simulink model "MPC_Validation"  (R2020a)
settings: Solver=FixedStepAuto  StartTime=0.0  StopTime=tsim  FixedStep=baseRate  RelTol=1e-3  EnableMultiTasking=on
values from neighbouring files (symbols this model uses):
  Ad = -C(7:12,4:9)    [theFastMPCSolver3.m]    (also in theInitializer.m = dss.A)
  ALGORITHM = 5    [Run_Initializer.m]
  baseRate = 0.05    [Run_Initializer.m]
  cdockdeltax = rc+rt-2*dockoffset    (= 0.165)    [theInitializer.m]
  cdockoa = atan(cdockdeltay/cdockdeltax)    [theInitializer.m]
  Cmat = zeros(6*N,9*N)    [theInitializer.m]
  con0 = [n*N, 2*N, N, N, N]    [Run_Initializer.m]
  drop_states_ARM = [ pi/2, pi/2, 0]    [Run_Initializer.m]
  drop_states_BLACK = rand([1,3])/10+init_states_BLACK    [Run_Initializer.m]
  drop_states_BLUE = rand([1,3])/10+init_states_BLUE    [Run_Initializer.m]
  drop_states_RED = rand([1,3])/10+init_states_RED    [Run_Initializer.m]
  ecoa = pi/2    (= 1.57079632679)    [theInitializer.m]
  F_Black_X_nominal = 0.2196    [Run_Initializer.m]
  F_Black_Y_nominal = 0.2825    [Run_Initializer.m]
  F_Blue_X_nominal = 0.2196    [Run_Initializer.m]
  F_Blue_Y_nominal = 0.2825    [Run_Initializer.m]
  F_red_X_nominal = 0.2196    [Run_Initializer.m]
  F_red_Y_nominal = 0.2825    [Run_Initializer.m]
  F_thrusters_BLACK = [F_Black_X_nominal; F_Black_X_nominal;                             F_Black_Y_nominal; F_Black_Y_nominal; F_Black_X_nominal;                              F_Black_X_nominal; F_Black_Y_nominal; F_Black_Y_nominal]    [Run_Initializer.m]
  F_thrusters_BLUE = [F_Blue_X_nominal; F_Blue_X_nominal;                             F_Blue_Y_nominal; F_Blue_Y_nominal; F_Blue_X_nominal;                              F_Blue_X_nominal; F_Blue_Y_nominal; F_Blue_Y_nominal]    [Run_Initializer.m]
  F_thrusters_RED = [F_red_X_nominal; F_red_X_nominal;                             F_red_Y_nominal; F_red_Y_nominal; F_red_X_nominal;                              F_red_X_nominal; F_red_Y_nominal; F_red_Y_nominal]    [Run_Initializer.m]
  Fmat = reshape(repmat([umax,umax,taumax],N,1),3*N,1)    [theInitializer.m]
  gamma = 0.95    [theInitializer.m]
  Gamma1 = 0.0025    [Run_Initializer.m]
  Gamma2 = 100    [Run_Initializer.m]
  Gamma3 = 10    [Run_Initializer.m]
  Gamma4 = 0.001    [Run_Initializer.m]
  Gamma5 = 100    [Run_Initializer.m]
  Gamma6 = 0.001    [Run_Initializer.m]
  H = blkdiag(pattern{:})    [theInitializer.m]
  home_states_BLACK = [ xLength/2, yLength/2, 0]    [Run_Initializer.m]
  home_states_BLUE = [ xLength/2-0.9, yLength/2+0.5, 0]    [Run_Initializer.m]
  home_states_RED = [ xLength/2+0.7, yLength/2, pi]    [Run_Initializer.m]
  init_states_BLACK = [ct;thetat0].'    [Run_Initializer.m]
  init_states_BLUE = [pobj1;0].'    [Run_Initializer.m]
  init_states_RED = xi(1:3).'    [Run_Initializer.m]
  isCONTROL = 0    [Run_Initializer.m]
  Kd_elarm = 0.05    [Run_Initializer.m]
  Kd_sharm = 0.05    [Run_Initializer.m]
  Kd_tb = 0.4    [Run_Initializer.m]
  Kd_tblue = 0.4    [Run_Initializer.m]
  Kd_tr = 0.4    [Run_Initializer.m]
  Kd_wrarm = 0.005    [Run_Initializer.m]
  Kd_xb = 8    [Run_Initializer.m]
  Kd_xblue = 8    [Run_Initializer.m]
  Kd_xr = 8    [Run_Initializer.m]
  Kd_yb = 8    [Run_Initializer.m]
  Kd_yblue = 8    [Run_Initializer.m]
  Kd_yr = 8    [Run_Initializer.m]
  KOZ_actual = KOZ + rc*sqrt(2)*1.1    [theInitializer.m]
  Kp = [0.08 0 0 ... (first row only)    [Run_Initializer.m]
  Kp_elarm = 0.08    [Run_Initializer.m]
  Kp_sharm = 0.15    [Run_Initializer.m]
  Kp_tb = 0.1    [Run_Initializer.m]
  Kp_tblue = 0.1    [Run_Initializer.m]
  Kp_tr = 0.1    [Run_Initializer.m]
  Kp_wrarm = 0.007    [Run_Initializer.m]
  Kp_xb = 2    [Run_Initializer.m]
  Kp_xblue = 2    [Run_Initializer.m]
  Kp_xr = 2    [Run_Initializer.m]
  Kp_yb = 2    [Run_Initializer.m]
  Kp_yblue = 2    [Run_Initializer.m]
  Kp_yr = 2    [Run_Initializer.m]
  Kv = [0.05 0 0 ... (first row only)    [Run_Initializer.m]
  maxiterations = 10    [Run_Initializer.m]
  N = 15    [Run_Initializer.m]    (also in theFastMPCSolver2.m = length(z)/9; theFastMPCSolver3.m = length(z)/9)
  n = size(b,1)    [my_fbsubstitution.m]    (also in theFastMPCSolver3.m)
  noise_variance_BLACK = 0    [Run_Initializer.m]
  noise_variance_BLUE = 0    [Run_Initializer.m]
  noise_variance_RED = 0    [Run_Initializer.m]
  noisemean = 0.1    [Run_Initializer.m]
  pdockoa = atan(rt/cdockdeltax)    [theInitializer.m]
  pdockr = sqrt(cdockdeltax*cdockdeltax + rt*rt)    [theInitializer.m]
  Phase0_End = Phase0_Duration    (= 5)    [Run_Initializer.m]
  Phase1_End = Phase0_Duration + Phase1_Duration    (= 10)    [Run_Initializer.m]
  Phase2_End = Phase0_Duration + Phase1_Duration +                                   Phase2_Duration    (= 36)    [Run_Initializer.m]
  Phase3_End = Phase0_Duration + Phase1_Duration +                                   Phase2_Duration + Phase3_Duration    (= 166)    [Run_Initializer.m]
  Phase3_SubPhase1_End = Phase2_End + Phase3_SubPhase1_Duration    (= 40)    [Run_Initializer.m]
  Phase3_SubPhase2_End = Phase2_End + Phase3_SubPhase1_Duration +                                   Phase3_SubPhase2_Duration    (= 42)    [Run_Initializer.m]
  Phase3_SubPhase3_End = Phase2_End + Phase3_SubPhase1_Duration +                                   Phase3_SubPhase2_Duration +                                  Phase3_SubPhase3_Duration    (= 44)    [Run_Initializer.m]
  Phase3_SubPhase4_End = Phase2_End + Phase3_SubPhase1_Duration +                                   Phase3_SubPhase2_Duration +                                  Phase3_SubPhase3_Duration +                                  Phase3_SubPhase4_Duration    [Run_Initializer.m]
  Phase4_End = Phase0_Duration + Phase1_Duration +                                   Phase2_Duration + Phase3_Duration +                                   Phase4_Duration    (= 186)    [Run_Initializer.m]
  Phase5_End = Phase0_Duration + Phase1_Duration +                                   Phase2_Duration + Phase3_Duration +                                   Phase4_Duration + Phase5_Duration    (= 191)    [Run_Initializer.m]
  rcone = 0.75    [theInitializer.m]
  rdock = sqrt(cdockdeltax*cdockdeltax + cdockdeltay*cdockdeltay)    [theInitializer.m]
  serverRate = 0.1    [Run_Initializer.m]
  Sj = [KOZ_actual^(-2),0; 0,KOZ_actual^(-2)]    [theInitializer.m]
  taumax = umax*rc    (= 0.0225)    [theInitializer.m]
  Td = 2    [Run_Initializer.m]
  thetah = 20.0 * d2r    (= 0.349065850399)    [theInitializer.m]
  thetat_dot = 0 * d2r    (= 0)    [Run_Initializer.m]
  thruster_dist2CG_BLACK = [83.42;-52.58;55.94;-60.05;54.08;-53.92;77.06;-55.94]    [Run_Initializer.m]
  thruster_dist2CG_BLUE = [73.54;-64.46;81.39;-60.11;64.46;-65.94;54.61;-74.39]    [Run_Initializer.m]
  thruster_dist2CG_RED = [49.92;-78.08;70.46;-63.54;81.08;-50.42;57.44;-75.96]    [Run_Initializer.m]
  tol = 0.00015    [Run_Initializer.m]
  Tz_lim_elarm = .1    (= 0.1)    [Run_Initializer.m]
  Tz_lim_sharm = .1    (= 0.1)    [Run_Initializer.m]
  Tz_lim_wrarm = .1    (= 0.1)    [Run_Initializer.m]
  Umat = zeros(3*N,9*N)    [theInitializer.m]
  umax = 0.15    [theInitializer.m]
  vobj1 = [0.00;0.00]    [Run_Initializer.m]
  vtar = [0.0;0.0]    [Run_Initializer.m]
undefined symbols (not defined in the file or in its folder): DiscIntNeverNeededParam, model_param, platformSelection, simMode, WhoAmI
libraries: dspstat3 x23, dspsigops x15, embdlinuxlib x10, raspberrypiBasiclib x10, simulink x8, MainLibrary x7, mspfiltlib x3, dsparch4 x3, dspswit3 x2, sensehatlib x1
(part 16 of 18)

== matlab function MPC_Validation/Triggered Subsystem/If Action Subsystem1/MPC ==
  data: CONTROL output; xi input; Td parameter; N parameter; pdockr parameter; rdock parameter; thetah parameter; KOZ_actual parameter; Sj parameter; rcone parameter; Ad parameter; con0 parameter; Cmat parameter; Umat parameter; Fmat parameter; H parameter; gamma parameter; tol parameter; x0 output; rhold output; x0 input; rhold input; ALGORITHM parameter; umax parameter; taumax parameter; n parameter; ct input; pobj1 input; vtar input; vobj1 input; thetat0 input; thetat_dot input; pdockoa parameter; ecoa parameter; cdockoa parameter; maxiterations parameter; CPUTIME output; cdockdeltax parameter
function [CONTROL, x0, rhold, CPUTIME] = MPC(xi,Td, N, pdockr, rdock, thetah, KOZ_actual, Sj, rcone, Ad, con0, Cmat, Umat, Fmat, H, gamma, tol, x0, rhold, ALGORITHM, umax, taumax, n, ct, pobj1, vtar, vobj1, thetat0, thetat_dot, pdockoa, ecoa, cdockoa, maxiterations, cdockdeltax)
    % COPY-PASTED FROM LOOP IN MAIN
    d2r = pi/180;
    
    N = 15;
    maxiterations = 10;
    
    % The moving target and obstacle positions for the current sampling instant, k
    [pobj1hz, ptar] = theMovingObstacleHorizonParameters(Td,N,ct,pobj1,vtar,vobj1);
    
    % The rotating target parameters for the current sampling instant, k
    [thetat,m1,m2,nc1,nc2,pdock,xt,cdock] = theRotatingTargetHorizonParameters(Td,N,ptar,vtar,pdockr,rhold,rdock,cdockoa,pdockoa,ecoa,thetat_dot,thetah,thetat0,cdockdeltax);
    
    % Reshape the xt variable for use in theObjectiveFunction, ignore the
    % current state and reform into [03 xt(2) 03 xt(2) 03 ... 03 xt(N+1)]
    xt9 = zeros(9,N);
    xt9(4:9,:) = xt(:,2:N+1);
    xt9 = reshape(xt9, [9*N,1]);
    
    % The reference trajectory of the chaser over the horizon of instant k
    pxref = theReferenceTrajectory(x0,N); % 2xN

    % The points ro on the KOZ boundaries of the obstacles over the horizon
    ro_1 = theObstacleLinearizer(pxref,pobj1hz(:,2:N+1),KOZ_actual);
    ro_t = theObstacleLinearizer(pxref,ptar(:,2:N+1),rhold);
    
    % Reshape pdock for use in the linearized matrix constraints
    pdock9 = zeros(9,N);
    pdock9(4:5,:) = pdock(:,2:N+1);
    pdock9 = reshape(pdock9, [9*N,1]);

    % Make the ro_X and robj9 vectors for obstacle constraints
    ro_1_9 = zeros(9,N);
    ro_1_9(4:5,:) = ro_1;
    ro_1_9 = reshape(ro_1_9,9*N,1);

    ro_t_9 = zeros(9,N);
    ro_t_9(4:5,:) = ro_t;
    ro_t_9 = reshape(ro_t_9,9*N,1);

    robj1_9 = zeros(9,N);
    robj1_9(4:5,:) = pobj1hz(:,2:N+1);
    robj1_9 = reshape(robj1_9,9*N,1);

    rtar_9 = zeros(9,N);
    rtar_9(4:5,:) = ptar(:,2:N+1);
    rtar_9 = reshape(rtar_9,9*N,1);

    % Make the matrix for obstacle constraints
    S1 = Sj;
    St = [1/(rhold*rhold), 0; 0, 1/(rhold*rhold)];

    E1 = (ro_1 - pobj1hz(:,2:N+1)).' * S1;
    Et = (ro_t - ptar(:,2:N+1)).' * St;

    D1 = zeros(N,(9*N));
    Dt = zeros(N,(9*N));
    for row = 1:N
        D1(row,4+(row-1)*9:5+(row-1)*9) = E1(row,:);
        Dt(row,4+(row-1)*9:5+(row-1)*9) = Et(row,:);
    end  
    
    % Define the b vector for Cx = b dynamics constraint
    bvec = zeros(6*N,1);
    bvec(1:6) = Ad*xi;
    
    % Define arrays for the hyperplane normal arrays to be used for the entry cone constraints
    nc1m = zeros(N,9*N);
    nc2m = zeros(N,9*N);
        
    % Determine if the entry cone constraints should be on
    if ((xi(1:2) - cdock(1:2,1)).' * (xi(1:2) - cdock(1:2,1)) < rcone*rcone) % if chaser is within rcone range
        
        temp1 = -nc1(2,:) * x0(4:5) + nc1(2,:) * pdock9(4:5);
        temp2 = nc2(2,:) * x0(4:5) - nc2(2,:) * pdock9(4:5);
        
              
        if temp1 <= 0 && temp2 <= 0 % only turn ec constraints on if it won't cause infeasibilities at the next step
            
        
            withEntryCone = 1; % turn on
            con = [n*N, 2*N, N, N, N, N, N];

            % Create Nx2N matrix of the entry cone normal to each hyperplane
            % Should be in the form
            % ncm = [ 0_1x3 n1_1x2 0_1x4 0_1x3  0_1x2 0_1x4  ... 0_1x3 0_1x2 0_1x4
            %         0_1x3  0_1x2 0_1x4 0_1x3 n2_1x2 0_1x4  ... 0_1x3 0_1x2 0_1x4
            %                           ...
            %         0_1x3  0_1x2 0_1x4 0_1x3  0_1x2 0_1x4  ... 0_1x3 nN+1_1x2 0_1x4
            for i=1:N
                nc1m(i,4+(i-1)*9:5+(i-1)*9) = nc1(i+1,:);
                nc2m(i,4+(i-1)*9:5+(i-1)*9) = nc2(i+1,:);
            end
        else
            
            withEntryCone = 0; % turn off
            con = con0;

            % FOR PLOTTING PURPOSES
            m1 = NaN;
            m2 = NaN;
        end
                
    else
        withEntryCone = 0; % turn off
        con = con0;
        
        % FOR PLOTTING PURPOSES
        m1 = NaN;
        m2 = NaN;
    end
    

    
%     if ALGORITHM == 5     
        % Constraint Matrix
        if ~withEntryCone
            Wmat = [-2*D1;-2*Dt];
        else
            Wmat = [-2*D1;-2*Dt;-nc1m;nc2m];
        end
%     % THIS NEEDS TO BE CLEANED UP
%     elseif ALGORITHM == 6 || ALGORITHM == 7
%         if withEntryCone
%             Wmat = zeros(10*N,9*N);
%             hvec = zeros(10*N,1);
%         else
%             Wmat = zeros(8*N,9*N);
%             hvec = zeros(8*N,1);
%         end
% 
%         for index = 0:N-1
%             blockc = 9*index;
%             if withEntryCone
%                 blockr = 10*index;
%                 Wmat(9+blockr,:) = -nc1m(index+1,:);
%                 Wmat(10+blockr,:) = nc2m(index+1,:);
%             else
%                 blockr = 8*index;
%             end
%             Wmat(1+blockr:3+blockr,1+blockc:3+blockc) = eye(3);
%             Wmat(4+blockr:6+blockr,1+blockc:3+blockc) = -eye(3);
%             Wmat(7+blockr,:) = -2*D1(index+1,:);
%             Wmat(8+blockr,:) = -2*Dt(index+1,:);
%         end
% 
%         f_D1 = -ones(N,1) - D1*(ro_1_9 + robj1_9);
%         f_Dt = -ones(N,1) - Dt*(ro_t_9 + rtar_9);   
%         if withEntryCone % if entry cone constraints turned on
%             f_ec1 = -nc1m * pdock9;
%             f_ec2 = nc2m * pdock9;
%         end
% 
%         for index = 0:N-1
%             if withEntryCone % if entry cone constraints turned on
%                 blockr = 10*index;
%                 hvec(9+blockr) = f_ec1(index+1);
%                 hvec(10+blockr) = f_ec2(index+1);
%             else
%                 blockr = 8*index;
%             end
% 
%             hvec(1+blockr:3+blockr) = [umax;umax;taumax];
%             hvec(4+blockr:6+blockr) = [umax;umax;taumax];
%             hvec(7+blockr) = f_D1(index+1);
%             hvec(8+blockr) = f_Dt(index+1);
%         end
% 
%     end
    
    % Constraint upper and lower limits
%     if ALGORITHM == 5
        [cl,cu,bineqvec] = theConstraintLimits4(Umat,Fmat,Wmat,con0,con,...
            D1,Dt,ro_1_9,ro_t_9,robj1_9,rtar_9,nc1m,...
            nc2m,pdock9);
%     end
    
    

%     
%     % Ensure a feasible start
%     if ALGORITHM == 6 || ALGORITHM == 7
%         if any((hvec - Wmat*x0) <= 0)
%             disp('Started with infeasible solution (outside).');
%             infeas0 = find((hvec - Wmat*x0) <= 0);
%             disp(infeas0)
% 
%             % Find a new feasible z-val for the violated constraint(s)
%             for ind = infeas0.'
%                 if size(con) == size(con0) % no ec constraints yet
%                     ind_startrange = 7 + 8*idivide(ind,int16(8+1));
%                     ind_endrange = ind_startrange + 1;
%                 else
%                     ind_startrange = 7 + 10*idivide(ind,int16(10+1));
%                     ind_endrange = ind_startrange + 3;
%                 end
% %                 disp(ind_startrange)
% %                 disp(ind_endrange)
%                     
%                 z_infeas_ind = find(Wmat(ind,:)); % optimization variable(s) to vary
%     %             disp('z(infeas)=')
%     %             disp(z_infeas_ind)
% 
%                 newind = z_infeas_ind - 9;
%                 
%                 search_range = 1;
%                 search_stepnum = 1001;
%                 
%                 while (1)
%                     if newind < 0
%                         disp("Sampling...")
% 
%                         % make a grid of search points
%                         try_x = linspace(x0(z_infeas_ind(1))-search_range,x0(z_infeas_ind(1))+search_range,search_stepnum);
%                         try_y = linspace(x0(z_infeas_ind(2))-search_range,x0(z_infeas_ind(2))+search_range,search_stepnum);
%                         [xx,yy] = meshgrid(try_x,try_y);
% 
%                         % calcuate the constraint at each grid point
% %                         temp = zeros(search_stepnum,search_stepnum);
%                         temp2 = zeros(search_stepnum*search_stepnum,3);
%                         for i1=1:search_stepnum
%                             for i2 = 1:search_stepnum
%                                 temp = hvec(ind_startrange:ind_endrange) - Wmat(ind_startrange:ind_endrange,z_infeas_ind)*[xx(i1,i2);yy(i1,i2)];
% 
%                                 % take note of grid points that satisfy the constraint
%                                 if ~any(temp <= 0)
%                                     temp2((i1-1)*search_stepnum+i2,1) = min(temp);
%                                     temp2((i1-1)*search_stepnum+i2,2) = i1;
%                                     temp2((i1-1)*search_stepnum+i2,3) = i2;
%                                 end
%                             end
%                         end
% 
%                         % get rid of data that does not satisfy the constraints
%                         temp2( ~any(temp2,2), : ) = [];  %rows
%                         
%                         if isempty(temp2)
%                             search_range = 3;
%                             search_stepnum = search_stepnum * 2;
%                             continue
%                         end
% 
%                         % choose one of the grid points that satisfy the constraint
%                         % currently finds the first minimum value... could be further improved
%                         ind_of_min = find(temp2(:,1) == min(temp2(:,1)));
%                         ind_chosen = ind_of_min(1);
% 
%                         % update the x0 with the new grid point
%                         [i1i2_chosen] = temp2(ind_chosen,[2,3]);
%                         i1_chosen = i1i2_chosen(1);
%                         i2_chosen = i1i2_chosen(2);
%                         x0(z_infeas_ind) = [xx(i1_chosen,i2_chosen);yy(i1_chosen,i2_chosen)];                     
%                         
%                     else
%                         x0(z_infeas_ind) = x0(newind); % re-tracing previous sol'n
%                     end
% 
%                     if (hvec(ind)- Wmat(ind,:)*x0) <= 0
%                         if newind < 0
%                             disp("Solution not in sample range.")
%                         else
%                             newind = newind - 9;
%                         end
%                     else
%                         disp("Resolved.")
%                         break
%                         
%                     end
%                 end
%             end
%         end
%        
%     end
%     
%     
%     
%     % Setup Options
%     if ALGORITHM == 5
        options = optimoptions('quadprog','Algorithm','active-set','MaxIterations',10);
%     elseif ALGORITHM == 6 || ALGORITHM == 7
%         nu = zeros(6*N,1);
%     end
%     
%     % Solve!
%     if ALGORITHM == 5
        tic
        [x,fval] = quadprog(H,-H.'*xt9,Wmat,bineqvec,Cmat,bvec,cl,cu,x0,options);
        CPUTIME = toc;
%     elseif ALGORITHM == 6
%         disp('----------------------------------------------')
%         disp(string(count))
%         
%         tic
%         [x,nu] = theFastMPCSolver2(x0,nu,xt9,H,Cmat,bvec,Wmat,hvec,1e-9,0.01,0.95,maxiterations);
%         solCPUtime = toc;
%     elseif ALGORITHM == 7
%         disp('----------------------------------------------')
%         disp(string(count))
%         tic
%         [x,nu] = theFastMPCSolver3(x0,nu,xt9,H,Cmat,bvec,Wmat,hvec,1e-9,0.01,0.95,maxiterations);
%         solCPUtime = toc;
%     end
   

    % Save data
%     sol(end+1:end+9) = x(1:9);
%     soliter(1:n,count) = xi;
%     soliter(n+1:n+9*N,count) = x;
%     solpobj(count,1) = pobj1hz(1,1); 
%     solpobj(count,2) = pobj1hz(2,1);
%     solpobj(count,3) = pobj2hz(1,1);
%     solpobj(count,4) = pobj2hz(2,1);
%     solptar(count,1) = ptar(1,1);
%     solptar(count,2) = ptar(2,1);
%     solm1(count,1) = m1(1);
%     solm2(count,1) = m2(1);
%     solthetat(count,1) = thetat(1);
%     solpdock(count,1:2) = pdock(:,1);
%     if ALGORITHM == 0
%         solJ(end+1) = theObjectiveFunction0(x,N,xt,P,Q,R);
%     elseif ALGORITHM > 0
%         solJ(end+1) = theObjectiveFunction123(x,xt9,H);
%     end
%     count = count + 1;

    CONTROL = x(1:3);
    
    % Determine if the chaser is docked using the 'current' positions of
    % the chaser and docking condition; done using only position
    if (xi(1:2) - cdock(1:2,1)).' * (xi(1:2) - cdock(1:2,1)) < tol
        isdocked = 1;
    end
    
    % Set the next guess as the solution from the previous iteration
    xi = x(4:9); % the next 'current' state of the chaser spacecraft
    % x0 = [x(10:end);0;0;0;Ad*x0(4+9*(N-2):9+9*(N-2)) + Bd*x0(1+9*(N-1):3+9*(N-1))];
    x0 = [x(10:end);0;0;0;x(4+9*(N-1):9+9*(N-1))];
    
    % Update rhold if:
    %  - the position of the chaser matches the holding position, within tolerance
    %  - the attitude of the chaser matches the docking condition, within tolerance
    %  - the holding radius is larger than its minimum allowable size, rdock
    if abs((xi(1:2) - xt(1:2,1)).' * (xi(1:2) - xt(1:2,1))) < 0.5 % if position error is below tolerance
        if abs(xi(3) - cdock(3,1)) < 10*d2r % if attitude error is below tolerance
            if rhold > rdock
                rhold = rhold * gamma; % decrease the holding radius
                if rhold < rdock
                    rhold = rdock; % set to the minimum holding radius, rdock
                end
            end
        end
    end
    
    % Set the next 'current' target and obstacle positions
%     ct = ptar(:,2);
%     pobj1 = pobj1hz(:,2); 
%     pobj2 = pobj2hz(:,2);
        
    % Set the new target theta value for the next iteration
%     thetat0 = thetat(2);
    
end

== matlab function MPC_Validation/Phase #3: Experiment/Change BLACK Behavior/Sub-Phase #2 /Hough Control/MATLAB Function2 ==
  data: Oy output; z input; Ox output
function [Oy, Ox]   = C3( z )
%C3 gives the rotation matrix about the z-axis for an angle 'z'
%   z - the angle about the z-axis which you rotate
%   A - the rotation matrix

Ox = [cos(z) sin(z); -sin(z) cos(z)]*[1;0];
Oy = [cos(z) sin(z); -sin(z) cos(z)]*[0;1];
end

== matlab function MPC_Validation/Phase #3: Experiment/Change BLACK Behavior/Sub-Phase #2 /Hough Control/MATLAB Function4 ==
  data: Oy input; e_out output; e_in input
function e_out = fcn(Oy, e_in)

a = sign(Oy'*e_in);
e_out = -a*norm(e_in);

== matlab function MPC_Validation/Phase #3: Experiment/Change BLACK Behavior/Sub-Phase #4/Hough Control/MATLAB Function4 ==
  data: Oy input; e_out output; e_in input
function e_out = fcn(Oy, e_in)

a = sign(Oy'*e_in);
e_out = -a*norm(e_in);

== matlab function MPC_Validation/Phase #3: Experiment/Change BLACK Behavior/Sub-Phase #1/Hough Control/MATLAB Function2 ==
  data: Oy output; z input; Ox output
function [Oy, Ox]   = C3( z )
%C3 gives the rotation matrix about the z-axis for an angle 'z'
%   z - the angle about the z-axis which you rotate
%   A - the rotation matrix

Ox = [cos(z) sin(z); -sin(z) cos(z)]*[1;0];
Oy = [cos(z) sin(z); -sin(z) cos(z)]*[0;1];
end

== matlab function MPC_Validation/Phase #3: Experiment/Change BLACK Behavior/Sub-Phase #1/Hough Control/MATLAB Function3 ==
  data: z input; Ox output
function Ox    = C3( z )
%C3 gives the rotation matrix about the z-axis for an angle 'z'
%   z - the angle about the z-axis which you rotate
%   A - the rotation matrix

Ox = [cos(z) sin(z); -sin(z) cos(z)]*[1;0];
end

== matlab function MPC_Validation/Phase #3: Experiment/Change BLACK Behavior/Sub-Phase #1/Hough Control/MATLAB Function4 ==
  data: Oy input; e_out output; e_in input
function e_out = fcn(Oy, e_in)

a = sign(Oy'*e_in);
e_out = -a*norm(e_in);

== matlab function MPC_Validation/Phase #3: Experiment/Change BLUE Behavior/Sub-Phase #4/Hough Control/MATLAB Function3 ==
  data: z input; Ox output
function Ox    = C3( z )
%C3 gives the rotation matrix about the z-axis for an angle 'z'
%   z - the angle about the z-axis which you rotate
%   A - the rotation matrix

Ox = [cos(z) sin(z); -sin(z) cos(z)]*[1;0];
end

== matlab function MPC_Validation/Phase #3: Experiment/Change BLUE Behavior/Sub-Phase #4/Hough Control/MATLAB Function4 ==
  data: Oy input; e_out output; e_in input
function e_out = fcn(Oy, e_in)

a = sign(Oy'*e_in);
e_out = -a*norm(e_in);

== matlab function MPC_Validation/Phase #5: Hold Home/Change BLACK Behavior/Hough Control/MATLAB Function2 ==
  data: Oy output; z input; Ox output
function [Oy, Ox]   = C3( z )
%C3 gives the rotation matrix about the z-axis for an angle 'z'
%   z - the angle about the z-axis which you rotate
%   A - the rotation matrix

Ox = [cos(z) sin(z); -sin(z) cos(z)]*[1;0];
Oy = [cos(z) sin(z); -sin(z) cos(z)]*[0;1];
end

== matlab function MPC_Validation/Phase #5: Hold Home/Change BLACK Behavior/Hough Control/MATLAB Function3 ==
  data: z input; Ox output
function Ox    = C3( z )
%C3 gives the rotation matrix about the z-axis for an angle 'z'
%   z - the angle about the z-axis which you rotate
%   A - the rotation matrix

Ox = [cos(z) sin(z); -sin(z) cos(z)]*[1;0];
end

== matlab function MPC_Validation/Phase #5: Hold Home/Change BLACK Behavior/Hough Control/MATLAB Function4 ==
  data: Oy input; e_out output; e_in input
function e_out = fcn(Oy, e_in)

a = sign(Oy'*e_in);
e_out = -a*norm(e_in);

== matlab function MPC_Validation/Phase #4: Return Home/Change BLUE Behavior/Hough Control/MATLAB Function2 ==
  data: Oy output; z input; Ox output
function [Oy, Ox]   = C3( z )
%C3 gives the rotation matrix about the z-axis for an angle 'z'
%   z - the angle about the z-axis which you rotate
%   A - the rotation matrix

Ox = [cos(z) sin(z); -sin(z) cos(z)]*[1;0];
Oy = [cos(z) sin(z); -sin(z) cos(z)]*[0;1];
end

== matlab function MPC_Validation/Phase #4: Return Home/Change BLUE Behavior/Hough Control/MATLAB Function3 ==
  data: z input; Ox output
function Ox    = C3( z )
%C3 gives the rotation matrix about the z-axis for an angle 'z'
%   z - the angle about the z-axis which you rotate
%   A - the rotation matrix

Ox = [cos(z) sin(z); -sin(z) cos(z)]*[1;0];
end

== matlab function MPC_Validation/Phase #4: Return Home/Change BLUE Behavior/Hough Control/MATLAB Function4 ==
  data: Oy input; e_out output; e_in input
function e_out = fcn(Oy, e_in)

a = sign(Oy'*e_in);
e_out = -a*norm(e_in);

== matlab function MPC_Validation/Simulate Plant Dynamics/BLUE Dynamics/BLUE  Dynamics Model/MATLAB Function ==
  data: control_inputs input; x_ddot output; model_param parameter
function x_ddot = BLUE_dynamics(control_inputs, model_param)

%#codegen
% Fully define the size of x_ddot() for code generation:
x_ddot     = zeros(3,1);

% Extract the servicer model parameters from the model_param vector defined
% in initialize.m:
m_BLUE    = model_param(5);
I_BLUE    = model_param(6);

% Extract the control inputs from the control_input vector:
Fx        = control_inputs(1);              % [N]
Fy        = control_inputs(2);              % [N]
Tz        = control_inputs(3);              % [N.m]

% Calculate the state acceleration vector:
x_ddot(1) = Fx/m_BLUE;                      % [m/s^2]
x_ddot(2) = Fy/m_BLUE;                      % [m/s^2]
x_ddot(3) = Tz/I_BLUE;                      % [rad/s^2]

end

== matlab function MPC_Validation/Phase #3: Experiment/Change BLUE Behavior/Sub-Phase #2 /Hough Control/MATLAB Function2 ==
  data: Oy output; z input; Ox output
function [Oy, Ox]   = C3( z )
%C3 gives the rotation matrix about the z-axis for an angle 'z'
%   z - the angle about the z-axis which you rotate
%   A - the rotation matrix

Ox = [cos(z) sin(z); -sin(z) cos(z)]*[1;0];
Oy = [cos(z) sin(z); -sin(z) cos(z)]*[0;1];
end

== matlab function MPC_Validation/Phase #3: Experiment/Change BLUE Behavior/Sub-Phase #2 /Hough Control/MATLAB Function3 ==
  data: z input; Ox output
function Ox    = C3( z )
%C3 gives the rotation matrix about the z-axis for an angle 'z'
%   z - the angle about the z-axis which you rotate
%   A - the rotation matrix

Ox = [cos(z) sin(z); -sin(z) cos(z)]*[1;0];
end

== matlab function MPC_Validation/Phase #3: Experiment/Change BLUE Behavior/Sub-Phase #2 /Hough Control/MATLAB Function4 ==
  data: Oy input; e_out output; e_in input
function e_out = fcn(Oy, e_in)

a = sign(Oy'*e_in);
e_out = -a*norm(e_in);

== matlab function MPC_Validation/Phase #5: Hold Home/Change BLUE Behavior/Hough Control/MATLAB Function2 ==
  data: Oy output; z input; Ox output
function [Oy, Ox]   = C3( z )
%C3 gives the rotation matrix about the z-axis for an angle 'z'
%   z - the angle about the z-axis which you rotate
%   A - the rotation matrix

Ox = [cos(z) sin(z); -sin(z) cos(z)]*[1;0];
Oy = [cos(z) sin(z); -sin(z) cos(z)]*[0;1];
end

== matlab function MPC_Validation/Phase #5: Hold Home/Change BLUE Behavior/Hough Control/MATLAB Function3 ==
  data: z input; Ox output
function Ox    = C3( z )
%C3 gives the rotation matrix about the z-axis for an angle 'z'
%   z - the angle about the z-axis which you rotate
%   A - the rotation matrix

Ox = [cos(z) sin(z); -sin(z) cos(z)]*[1;0];
end

== matlab function MPC_Validation/Phase #5: Hold Home/Change BLUE Behavior/Hough Control/MATLAB Function4 ==
  data: Oy input; e_out output; e_in input
function e_out = fcn(Oy, e_in)

a = sign(Oy'*e_in);
e_out = -a*norm(e_in);

== matlab function MPC_Validation/From Torque Command RW/Change RED Behavior/Calculate Saturated RPM Signal/Calculate RW RPM Increment ==
  data: Tz_Sat input; dRPM_RW output
function dRPM_RW = Calc_RW_RPM(Tz_Sat)

dRPM_RW =  (Tz_Sat/0.007244720)*(60/2/pi)*0.1;

end

== matlab function MPC_Validation/From Torque Command RW/Change RED Behavior/Wheel RPM to PWM/Check if RW is Ready ==
  data: Status input; EnableSig output; WheelRPM_In input; WheelRPM_Out output
function [EnableSig, WheelRPM_Out] = Check_Wheel_Status(Status, WheelRPM_In)

if Status == 0
    EnableSig    = 1;
    WheelRPM_Out = WheelRPM_In;
else
    EnableSig    = 0;
    WheelRPM_Out = 0;
end

end

== matlab function MPC_Validation/From Torque Command RW/Change RED Behavior/Wheel RPM to PWM/Get RW Direction ==
  data: MotorRPM_Sat input; WheelDirection output
function WheelDirection = GetDirection(MotorRPM_Sat)

if MotorRPM_Sat > 0
    WheelDirection = 0;
else
    WheelDirection = 1;
end
        
end

== matlab function MPC_Validation/From Torque Command RW/Change RED Behavior/Wheel RPM to PWM/RPM to PWM Value ==
  data: MotorRPM_Sat input; MotorPWM output
function MotorPWM = RPM2PWM(MotorRPM_Sat)

PWMRange = 0.9-0.1;

MotorPWM = ((MotorRPM_Sat*PWMRange)/7000) + 0.1;

end

== matlab function MPC_Validation/Simulate Plant Dynamics/RED and ARM Dynamics/RED Only/RED Dynamics/RED Dynamics Model/MATLAB Function ==
  data: control_inputs input; x_ddot output; model_param parameter
function x_ddot = RED_dynamics(control_inputs, model_param)

%#codegen
% Fully define the size of x_ddot() for code generation:
x_ddot     = zeros(3,1);

% Extract the servicer model parameters from the model_param vector defined
% in initialize.m:
m_RED    = model_param(1);
I_RED    = model_param(2);

% Extract the control inputs from the control_input vector:
Fx        = control_inputs(1);              % [N]
Fy        = control_inputs(2);              % [N]
Tz        = control_inputs(3);              % [N.m]

% Calculate the state acceleration vector:
x_ddot(1) = Fx/m_RED;                      % [m/s^2]
x_ddot(2) = Fy/m_RED;                      % [m/s^2]
x_ddot(3) = Tz/I_RED;                      % [rad/s^2]

end

== matlab function MPC_Validation/Phase #3: Experiment/Change BLACK Behavior/Sub-Phase #3 /Hough Control/MATLAB Function2 ==
  data: Oy output; z input; Ox output
function [Oy, Ox]   = C3( z )
%C3 gives the rotation matrix about the z-axis for an angle 'z'
%   z - the angle about the z-axis which you rotate
%   A - the rotation matrix

Ox = [cos(z) sin(z); -sin(z) cos(z)]*[1;0];
Oy = [cos(z) sin(z); -sin(z) cos(z)]*[0;1];
end

== matlab function MPC_Validation/Phase #3: Experiment/Change BLACK Behavior/Sub-Phase #3 /Hough Control/MATLAB Function3 ==
  data: z input; Ox output
function Ox    = C3( z )
%C3 gives the rotation matrix about the z-axis for an angle 'z'
%   z - the angle about the z-axis which you rotate
%   A - the rotation matrix

Ox = [cos(z) sin(z); -sin(z) cos(z)]*[1;0];
end

== matlab function MPC_Validation/Phase #3: Experiment/Change BLUE Behavior/Sub-Phase #3 /Hough Control/MATLAB Function2 ==
  data: Oy output; z input; Ox output
function [Oy, Ox]   = C3( z )
%C3 gives the rotation matrix about the z-axis for an angle 'z'
%   z - the angle about the z-axis which you rotate
%   A - the rotation matrix

Ox = [cos(z) sin(z); -sin(z) cos(z)]*[1;0];
Oy = [cos(z) sin(z); -sin(z) cos(z)]*[0;1];
end

== matlab function MPC_Validation/IMU Data and Algorithms/Change RED Behavior/Create Rotation Matrix ==
  data: Rz input; C_Ib output
function C_Ib = RotateFrame(Rz)

C_bI = [  cos(Rz) sin(Rz)
         -sin(Rz) cos(Rz) ];

C_Ib = inv(C_bI);

end

== matlab function MPC_Validation/IMU Data and Algorithms/Change BLACK Behavior/Create Rotation Matrix ==
  data: Rz input; C_Ib output
function C_Ib = RotateFrame(Rz)

C_bI = [  cos(Rz) sin(Rz)
         -sin(Rz) cos(Rz) ];

C_Ib = inv(C_bI);

end

== matlab function MPC_Validation/IMU Data and Algorithms/Change RED Behavior/ChangeOrientation ==
  data: u input; y output
function y = ChangeOrientation(u)

y = rotz(-90)*u';

== matlab function MPC_Validation/IMU Data and Algorithms/Change BLACK Behavior/ChangeOrientation ==
  data: u input; y output
function y = ChangeOrientation(u)

y = rotz(-90)*u';

== matlab function MPC_Validation/IMU Data and Algorithms/Change BLUE Behavior/ChangeOrientation ==
  data: u input; y output
function y = ChangeOrientation(u)

y = rotz(-90)*u';

== matlab function MPC_Validation/IMU Data and Algorithms/Change BLUE Behavior/Create Rotation Matrix ==
  data: Rz input; C_Ib output
function C_Ib = RotateFrame(Rz)

C_bI = [  cos(Rz) sin(Rz)
         -sin(Rz) cos(Rz) ];

C_Ib = inv(C_bI);

end

== matlab function MPC_Validation/From Force//Torque to PWM Signal/Change RED Behavior/Calculate Thruster ON//OFF/MATLAB Function ==
  data: H output; thruster_dist2CG_RED parameter; F_thrusters_RED parameter; theta_1 input; theta_2 input; theta_3 input; model_param parameter
function H   = MakeHWithArm(thruster_dist2CG_RED,F_thrusters_RED, theta_1, theta_2, theta_3, model_param)

m0  = model_param(1);          
phi = model_param(7);
b0  = model_param(8);
a1  = model_param(9);
b1  = model_param(10);              
a2  = model_param(11);                
b2  = model_param(12);               
a3  = model_param(13);                         
m1  = model_param(15);
m2  = model_param(16);
m3  = model_param(17);

link1_com_x = b0*cos(phi) + a1*cos(pi/2 + theta_1);
link1_com_y = b0*sin(phi) + a1*sin(pi/2 + theta_1);

link2_com_x = link1_com_x + b1*cos(pi/2 + theta_1) + a2*cos(pi/2 + theta_1 + theta_2);
link2_com_y = link1_com_y + b1*sin(pi/2 + theta_1) + a2*sin(pi/2 + theta_1 + theta_2);

link3_com_x = link2_com_x + b2*cos(pi/2 + theta_1 + theta_2) + a3*cos(pi/2 + theta_1 + theta_2 + theta_3);
link3_com_y = link2_com_y + b2*sin(pi/2 + theta_1 + theta_2) + a3*sin(pi/2 + theta_1 + theta_2 + theta_3);

delta_com_due_to_arm_x = (m1*link1_com_x + m2*link2_com_x + m3*link3_com_x)/(m0 + m1 + m2 + m3)*1000; % [mm]
delta_com_due_to_arm_y = (m1*link1_com_y + m2*link2_com_y + m3*link3_com_y)/(m0 + m1 + m2 + m3)*1000; % [mm]

adjusted_thruster_dist2CG_RED = [thruster_dist2CG_RED(1)-delta_com_due_to_arm_y;
                                 thruster_dist2CG_RED(2)-delta_com_due_to_arm_y;
                                 thruster_dist2CG_RED(3)-delta_com_due_to_arm_x;
                                 thruster_dist2CG_RED(4)-delta_com_due_to_arm_x;
                                 thruster_dist2CG_RED(5)+delta_com_due_to_arm_y;
                                 thruster_dist2CG_RED(6)+delta_com_due_to_arm_y;
                                 thruster_dist2CG_RED(7)+delta_com_due_to_arm_x;
                                 thruster_dist2CG_RED(8)+delta_com_due_to_arm_x];
                                 


Vec1 = [ -1
         -1
          0 
          0
          1
          1
          0
          0 ];
      
Vec2 = [  0
          0
          1
          1
          0
          0
         -1
         -1 ];
     
Vec3 = adjusted_thruster_dist2CG_RED./1000;

Mat1 = [Vec1, Vec2, Vec3]';

Mat2 = diag((F_thrusters_RED./2));

H    = Mat1*Mat2;

end

== matlab function MPC_Validation/From Force//Torque to PWM Signal/Change RED Behavior/Calculate Thruster ON//OFF/MATLAB Function1 ==
  data: H output; thruster_dist2CG_RED parameter; F_thrusters_RED parameter
function H = MakeH(thruster_dist2CG_RED,F_thrusters_RED)

Vec1 = [ -1
         -1
          0 
          0
          1
          1
          0
          0 ];
      
Vec2 = [  0
          0
          1
          1
          0
          0
         -1
         -1 ];
     
Vec3 = thruster_dist2CG_RED./1000;

Mat1 = [Vec1, Vec2, Vec3]';

Mat2 = diag((F_thrusters_RED));

H    = Mat1*Mat2;

end

== matlab function MPC_Validation/Simulate Plant Dynamics/BLACK Dynamics/BLACK Dynamics Model/MATLAB Function ==
  data: control_inputs input; x_ddot output; model_param parameter
function x_ddot = BLACK_dynamics(control_inputs, model_param)

%#codegen
% Fully define the size of x_ddot() for code generation:
x_ddot     = zeros(3,1);

% Extract the servicer model parameters from the model_param vector defined
% in initialize.m:
m_BLACK    = model_param(3);
I_BLACK    = model_param(4);

% Extract the control inputs from the control_input vector:
Fx        = control_inputs(1);              % [N]
Fy        = control_inputs(2);              % [N]
Tz        = control_inputs(3);              % [N.m]

% Calculate the state acceleration vector:
x_ddot(1) = Fx/m_BLACK;                      % [m/s^2]
x_ddot(2) = Fy/m_BLACK;                      % [m/s^2]
x_ddot(3) = Tz/I_BLACK;                      % [rad/s^2]

end

== matlab function MPC_Validation/From Force//Torque to PWM Signal/Change RED Behavior/Calculate Thruster ON//OFF/MATLAB Function2 ==
  data: ThrustPer_Final output; ThrustPer input
function ThrustPer_Final  = ThrusterSat(ThrustPer)

ValveTime       = 0.007;
TControl        = 0.1;
ThrustPer_Final = zeros(8,1);

if max(ThrustPer) > 1
    ThrustPer_Sat = ThrustPer/max(ThrustPer);
else
    ThrustPer_Sat = ThrustPer;
end

for i = 1:8
    if ThrustPer_Sat(i) > ValveTime/TControl 
        ThrustPer_Final(i) = ThrustPer_Sat(i);
    else
        ThrustPer_Final(i) = 0;
    end
end
   

end

== matlab function MPC_Validation/From Force//Torque to PWM Signal/Change RED Behavior/Calculate Thruster ON//OFF/Rotate Forces to Inertial/Create Rotation Matrix ==
  data: Rz input; C_Ib output
function C_Ib = RotateFrame(Rz)

C_bI = [  cos(Rz) sin(Rz)
         -sin(Rz) cos(Rz) ];

C_Ib = inv(C_bI);

end

== matlab function MPC_Validation/Phase #3: Experiment/Change RED Behavior/Sub-Phase #4/RED+ARM/Transpose Jacobian Controller/Error Signal/End-Effector Position1 ==
  data: y output; q input; u input
function y = ForwardKinematics(q, u)
%#codegen
theta = q(3);

C_bI_RED = [  cos(theta) sin(theta)
            -sin(theta) cos(theta) ];
                                 
y  = C_bI_RED*u;  
end

== matlab function MPC_Validation/Phase #3: Experiment/Change BLACK Behavior/Sub-Phase #2 /Hough Control/MATLAB Function3 ==
  data: z input; Ox output
function Ox    = C3( z )
%C3 gives the rotation matrix about the z-axis for an angle 'z'
%   z - the angle about the z-axis which you rotate
%   A - the rotation matrix

Ox = [cos(z) sin(z); -sin(z) cos(z)]*[1;0];
end

== matlab function MPC_Validation/Simulate Plant Dynamics/RED and ARM Dynamics/RED + ARM/RED + ARM Dynamics/Coriolis Function ==
  data: x input; CoriolisS output; model_param parameter
function CoriolisS = CoriolisFunc3LINK(x, model_param)
%CORIOLISFUNC3LINK
%    CORIOLISS = CORIOLISFUNC3LINK(A1,A2,A3,B0,B1,B2,M1,M2,M3,PHI,Q0,Q1,Q2,Q3,Q0_DOT,Q1_DOT,Q2_DOT,Q3_DOT)

%    This function was generated by the Symbolic Math Toolbox version 8.5.
%    15-Mar-2022 15:58:58
q0 = x(3);
q1 = x(4);
q2 = x(5);
q3 = x(6);

q0_dot = x(9);
q1_dot = x(10);
q2_dot = x(11);
q3_dot = x(12);

m0= model_param(1);                  % RED Mass
I0= model_param(2);                  % RED Inertia;
phi= model_param(7);                 % ARM Phi
b0= model_param(8);                  % ARM b0
a1= model_param(9);                  % ARM a1
b1= model_param(10);                 % ARM b1
a2= model_param(11);                 % ARM a2
b2= model_param(12);                 % ARM b2
a3= model_param(13);                 % ARM a3
b3= model_param(14);                 % ARM b3
m1= model_param(15);                 % ARM m1
m2= model_param(16);                 % ARM m2
m3= model_param(17);                 % ARM m3
I1= model_param(18);                 % ARM I1
I2= model_param(19);                 % ARM I2
I3= model_param(20);                 % ARM I3

t2 = sin(q2);
t3 = sin(q3);
t4 = a1+b1;
t5 = a2+b2;
t6 = a1.*m1;
t7 = a2.*m2;
t8 = b0.*m1;
t9 = b0.*m2;
t10 = b0.*m3;
t11 = a1.*q0_dot;
t12 = a1.*q1_dot;
t13 = a2.*q0_dot;
t14 = a2.*q1_dot;
t15 = a2.*q2_dot;
t16 = b1.*q0_dot;
t17 = b1.*q1_dot;
t18 = b2.*q0_dot;
t19 = b2.*q1_dot;
t20 = b2.*q2_dot;
t21 = phi+q0;
t22 = q2+q3;
t23 = a3.*m3.*q0_dot;
t24 = a3.*m3.*q1_dot;
t25 = a3.*m3.*q2_dot;
t26 = a3.*m3.*q3_dot;
t28 = -phi;
t29 = -q1;
t71 = q0_dot+q1_dot+q2_dot+q3_dot;
t72 = pi./2.0;
t27 = sin(t22);
t30 = b0.*q0_dot.*t6;
t31 = b0.*q1_dot.*t6;
t32 = t9.*t11;
t33 = t9.*t12;
t34 = t10.*t11;
t35 = b0.*q0_dot.*t7;
t36 = t10.*t12;
t37 = b0.*q1_dot.*t7;
t38 = t10.*t13;
t39 = t7.*t16;
t40 = b2.*m3.*t11;
t41 = b0.*q2_dot.*t7;
t42 = t10.*t14;
t43 = t7.*t17;
t44 = b1.*m3.*t13;
t45 = a3.*q0_dot.*t10;
t46 = b2.*m3.*t12;
t47 = t10.*t15;
t48 = b1.*q2_dot.*t7;
t49 = b1.*m3.*t14;
t50 = a3.*q1_dot.*t10;
t51 = a3.*m3.*t16;
t52 = a1.*m3.*t20;
t53 = b1.*m3.*t15;
t54 = a3.*q2_dot.*t10;
t55 = a3.*m3.*t17;
t56 = a3.*q3_dot.*t10;
t57 = b1.*t25;
t58 = b1.*t26;
t59 = b2.*t26;
t60 = t9.*t16;
t61 = t9.*t17;
t62 = t10.*t16;
t63 = t10.*t17;
t64 = t10.*t18;
t65 = t10.*t19;
t66 = b2.*m3.*t16;
t67 = t10.*t20;
t68 = b2.*m3.*t17;
t69 = b1.*m3.*t20;
t70 = q0+q1+t22;
t73 = m2.*t4;
t74 = m3.*t4;
t75 = m3.*t5;
t76 = t7.*t11;
t77 = t7.*t12;
t78 = a2.*m3.*t11;
t79 = a1.*q2_dot.*t7;
t80 = a2.*m3.*t12;
t81 = a3.*m3.*t11;
t82 = a1.*m3.*t15;
t83 = a3.*m3.*t12;
t84 = a1.*t25;
t85 = a1.*t26;
t86 = a2.*t26;
t87 = -t23;
t88 = -t24;
t89 = -t25;
t90 = -t26;
t91 = phi+t29;
t128 = q1+q2+t28;
t140 = a3.*m3.*t71;
t142 = q1+t22+t28;
t143 = q0+q1+t72;
t152 = t8+t9+t10;
t161 = t11+t12+t16+t17;
t180 = t13+t14+t15+t18+t19+t20;
t92 = -t31;
t93 = -t33;
t94 = -t35;
t95 = -t36;
t96 = -t37;
t97 = -t38;
t98 = -t39;
t99 = -t40;
t100 = -t41;
t101 = -t42;
t102 = -t43;
t103 = -t44;
t104 = -t45;
t105 = -t46;
t106 = -t47;
t107 = -t48;
t108 = -t49;
t109 = -t50;
t110 = -t51;
t111 = -t52;
t112 = -t53;
t113 = -t54;
t114 = -t55;
t115 = -t56;
t116 = -t57;
t117 = -t58;
t118 = -t59;
t119 = -t61;
t120 = -t63;
t121 = -t64;
t122 = -t65;
t123 = -t66;
t124 = -t67;
t125 = -t68;
t126 = -t69;
t127 = cos(t91);
t129 = -t76;
t130 = -t77;
t131 = -t78;
t132 = -t79;
t133 = -t80;
t134 = -t81;
t135 = -t82;
t136 = -t83;
t137 = -t84;
t138 = -t85;
t139 = -t86;
t141 = cos(t128);
t144 = cos(t143);
t145 = q2+t143;
t146 = sin(t143);
t147 = t7+t75;
t148 = cos(t142);
t150 = t70+t72;
t158 = a3.*t71.*t74;
t159 = a3.*t71.*t75;
t160 = q0_dot.*t152;
t167 = t6+t73+t74;
t173 = a3.*m3.*t161;
t174 = t35+t38+t64;
t179 = -t3.*(t59+t86);
t181 = t51+t55+t81+t83;
t183 = a3.*m3.*t180;
t185 = t87+t88+t89+t90;
t190 = -t27.*(t57+t58+t84+t85);
t197 = -t2.*(t48+t52+t53+t69+t79+t82);
t203 = t39+t40+t43+t44+t46+t49+t66+t68+t76+t77+t78+t80;
t149 = cos(t145);
t151 = sin(t145);
t153 = cos(t150);
t154 = sin(t150);
t155 = q0_dot.*t147;
t156 = q1_dot.*t147;
t157 = q2_dot.*t147;
t165 = -t158;
t166 = -t159;
t168 = -t160;
t169 = t45.*t148;
t170 = t118+t139;
t171 = q0_dot.*t167;
t172 = q1_dot.*t167;
t182 = t27.*t173;
t184 = t141.*t174;
t186 = t3.*t183;
t187 = t27.*t181;
t188 = t116+t117+t137+t138;
t189 = t104+t109+t113+t115;
t194 = -t148.*(t45+t50+t54+t56);
t196 = t107+t111+t112+t126+t132+t135;
t204 = -t27.*(t57+t58+t84+t85+t181);
t205 = t94+t96+t97+t100+t101+t106+t121+t122+t124;
t206 = t2.*t203;
t207 = -t141.*(t37+t41+t42+t47+t65+t67+t174);
t209 = -t2.*(t48+t52+t53+t69+t79+t82+t203);
t162 = -t155;
t163 = -t156;
t164 = -t157;
t175 = t3.*t166;
t176 = -t171;
t177 = -t172;
t178 = t27.*t165;
t191 = -t153.*(t23+t24+t25+t26);
t192 = -t154.*(t23+t24+t25+t26);
t198 = -t144.*(t171+t172);
t199 = -t146.*(t171+t172);
t200 = -t149.*(t155+t156+t157);
t201 = -t151.*(t155+t156+t157);
t202 = t110+t114+t134+t136+t188;
t208 = t98+t99+t102+t103+t105+t108+t123+t125+t129+t130+t131+t133+t196;
t193 = t176+t177;
t195 = t162+t163+t164;
CoriolisS = reshape([0.0,0.0,0.0,0.0,0.0,0.0,0.0,0.0,0.0,0.0,0.0,0.0,t191+t198+t200+t168.*cos(t21),t192+t199+t201+t168.*sin(t21),t179+t190+t197-t127.*(t31+t33+t36+t61+t63)-t148.*(t50+t54+t56)-t141.*(t37+t41+t42+t47+t65+t67),t169+t179+t184+t190+t197+t127.*(t30+t32+t34+t60+t62),t169+t179+t184+t187+t206,t169+t182+t186,t191+t198+t200,t192+t199+t201,t179+t190+t194+t197+t207-t127.*(t30+t31+t32+t33+t34+t36+t60+t61+t62+t63),t179+t190+t197,t179+t187+t206,t182+t186,t191+t200,t192+t201,t179+t194+t204+t207+t209,t179+t204+t209,t3.*t5.*t90,a3.*t3.*t75.*(q0_dot+q1_dot+q2_dot),t140.*sin(t70),-t140.*cos(t70),t175+t178-a3.*t10.*t71.*t148,t175+t178,t175,0.0],[6,6]);

end

== matlab function MPC_Validation/Simulate Plant Dynamics/RED and ARM Dynamics/RED + ARM/RED + ARM Dynamics/Dynamics Model ==
  data: xdot output; x input; InertiaS input; CoriolisS input; u input; Gamma1 parameter; Gamma2 parameter; Gamma3 parameter; Gamma5 parameter; Gamma4 parameter; Gamma6 parameter
function xdot  = DynamicsModel(x, InertiaS, CoriolisS, u, Gamma1, Gamma2, Gamma3, Gamma5, Gamma4, Gamma6)

fqdot1 = Gamma1*(tanh(Gamma2*x(10)) - tanh(Gamma3*x(10))) + Gamma4*tanh(Gamma5*x(10)) + Gamma6*x(10);
fqdot2 = Gamma1*(tanh(Gamma2*x(11)) - tanh(Gamma3*x(11))) + Gamma4*tanh(Gamma5*x(11)) + Gamma6*x(11);
fqdot3 = Gamma1*(tanh(Gamma2*x(12)) - tanh(Gamma3*x(12))) + Gamma4*tanh(Gamma5*x(12)) + Gamma6*x(12);

q_ddot = pinv(InertiaS)*(u - CoriolisS*x(7:12) - [0;0;0;fqdot1;fqdot2;fqdot3]);

xdot   = [ x(7:12)
           q_ddot   ];
       
end
